simulink model "government"  (R2020a)
settings: Solver=VariableStepAuto  StartTime=0.0  StopTime=10.0  RelTol=1e-3
values from neighbouring files (symbols this model uses):
  sigma = 0.3    [main.m]
undefined symbols (not defined in the file or in its folder): target, Tf, Tg, To, Tp, tx, VAT
settings Model: Creator=erlended  LastModifiedBy=erlended

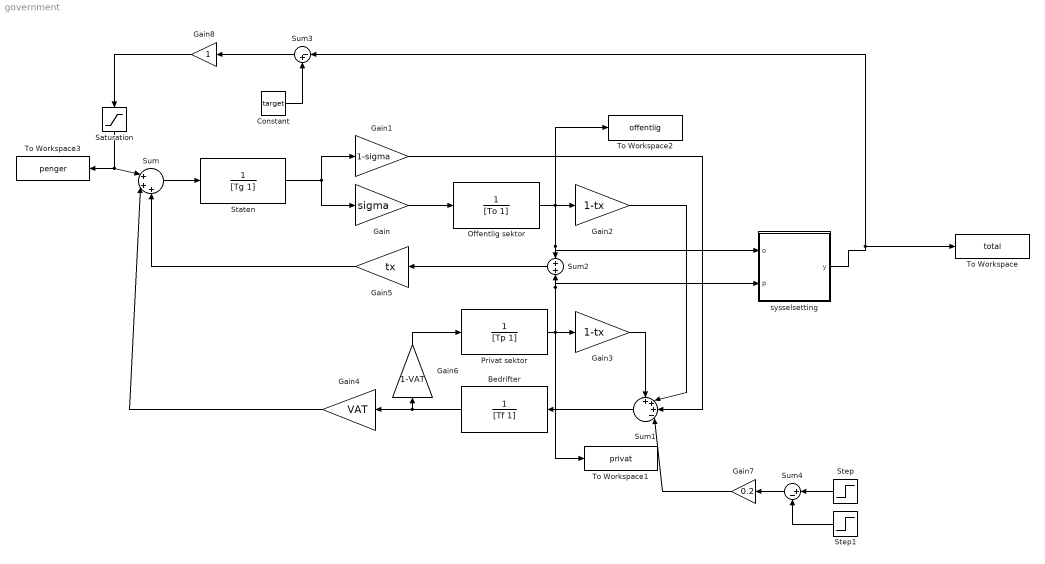
== system government ==
  Bedrifter : TransferFcn  Denominator=[Tf 1]
  Constant : Constant  Value=target
  Gain : Gain  Gain=sigma
  Gain1 : Gain  Gain=1-sigma
  Gain2 : Gain  Gain=1-tx
  Gain3 : Gain  Gain=1-tx
  Gain4 : Gain  Gain=VAT
  Gain5 : Gain  Gain=tx
  Gain6 : Gain  Gain=1-VAT
  Gain7 : Gain  Gain=0.2
  Gain8 : Gain
  Offentlig sektor : TransferFcn  Denominator=[To 1]
  Privat sektor : TransferFcn  Denominator=[Tp 1]
  Saturation : Saturate  UpperLimit=1  LowerLimit=0
  Staten : TransferFcn  Denominator=[Tg 1]
  Step : Step  Time=30  SampleTime=0
  Step1 : Step  Time=40  SampleTime=0
  Sum : Sum  Inputs=|+++
  Sum1 : Sum  Inputs=+++-|
  Sum2 : Sum  Inputs=+|+
  Sum3 : Sum  Inputs=|-+
  Sum4 : Sum  Inputs=|+-
  To Workspace : ToWorkspace  VariableName=total  SaveFormat=Timeseries  SampleTime=-1
  To Workspace1 : ToWorkspace  VariableName=privat  SaveFormat=Timeseries  SampleTime=-1
  To Workspace2 : ToWorkspace  VariableName=offentlig  SaveFormat=Timeseries  SampleTime=-1
  To Workspace3 : ToWorkspace  VariableName=penger  SaveFormat=Timeseries  SampleTime=-1
  sysselsetting : MATLAB Function  TreatAsAtomicUnit=on
  wires:
  Sum/1 -> Staten/1
  Staten/1 -> Gain/1, Gain1/1
  Gain/1 -> Offentlig sektor/1
  Gain2/1 -> Sum1/2
  Offentlig sektor/1 -> To Workspace2/1, sysselsetting/1(o), Sum2/1, Gain2/1
  Gain1/1 -> Sum1/3
  Privat sektor/1 -> To Workspace1/1, Gain3/1, sysselsetting/2(p), Sum2/2
  Gain3/1 -> Sum1/1
  Sum1/1 -> Bedrifter/1
  Bedrifter/1 -> Gain6/1, Gain4/1
  Gain4/1 -> Sum/2
  Sum2/1 -> Gain5/1
  Gain5/1 -> Sum/3
  Gain6/1 -> Privat sektor/1
  sysselsetting/1(y) -> Sum3/1, To Workspace/1
  Constant/1 -> Sum3/2
  Gain7/1 -> Sum1/4
  Sum3/1 -> Gain8/1
  Step/1 -> Sum4/1
  Sum4/1 -> Gain7/1
  Step1/1 -> Sum4/2
  Saturation/1 -> To Workspace3/1, Sum/1
  Gain8/1 -> Saturation/1

== matlab function government/sysselsetting ==
  data: o input; y output; p input
function  y= fcn(o, p)
salary = 1; 
employment = (o+p)/salary;

u = employment;

y = u;
